simulink library "lib_fuel_converter3"  (Simulink 4.1.1)
values from neighbouring files (symbols this model uses):
  logFlag = 1    [advSACompMaskInit.m]    (also in advSACompMaskInitR13.m)
undefined symbols (not defined in the file or in its folder): air_cp, amb_tmp, cyc_mph, ex_gas_cp, fc_acc_mass, fc_base_mass, fc_c2i_th_cond, fc_c_init_tmp, fc_cl2h_eff, fc_CO2_to_FUELgps, fc_cold, fc_cold_tmp, fc_cp, fc_ct_trq, fc_emisv, fc_ext_sarea, fc_fuel_den, fc_fuel_lhv, fc_h2x_th_cond, fc_h_air_flow, fc_h_cp, fc_h_init_tmp, fc_hood_emisv, fc_hood_sarea, fc_i2x_th_cond, fc_i_init_tmp, fc_inertia, fc_map_spd, fc_map_trq, fc_max_trq, fc_nn_model_name, fc_pwr_scale, fc_spd_scale, fc_trq_scale, fc_tstat, fc_x_init_tmp, fd_ratio, gb_num_init, gb_ratio, generalName, pow, vc_idle_bool, vc_idle_spd, vc_key_on, veh_glider_mass, wh_radius
libraries: lib_fuel_converter3 x4, lib_etc x4, lib_fuel_converter x2, lib_fuel_converter2 x1
(part 6 of 9)

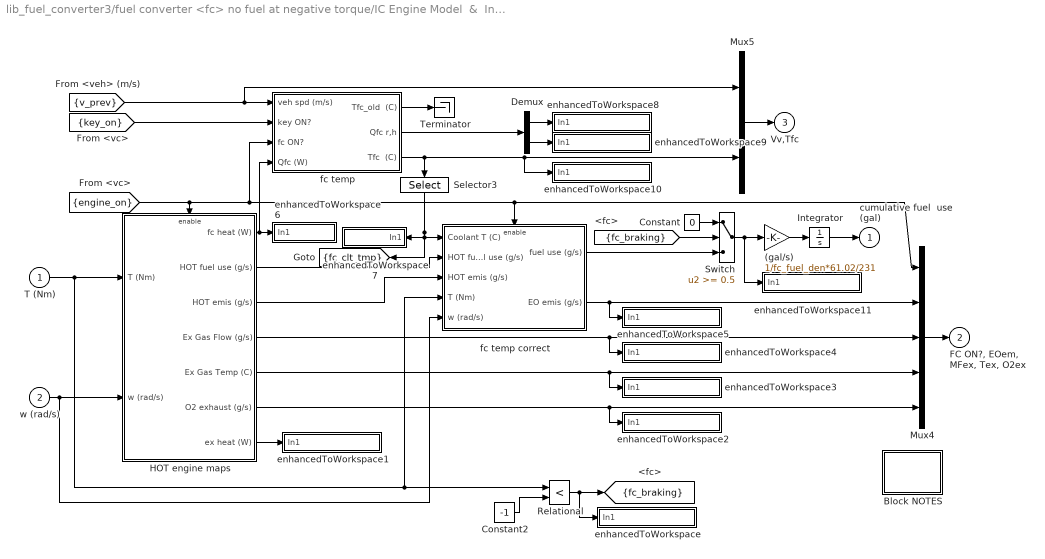
== system lib_fuel_converter3/fuel converter <fc> no fuel at negative torque/IC Engine Model  &  Interface/ic engine model/fuel use and EO emis no fuel used at negative torque ==
  T (Nm) : Inport  Port=1  LatchInput=off
  w (rad/s) : Inport  Port=2  LatchInput=off
  (gal/s) : Gain  Gain=1/fc_fuel_den*61.02/231  Multiplication=Element-wise(K.*u)  SaturateOnIntegerOverflow=on
  Block NOTES : Subsystem
      settings: RTWFcnNameOpts=Auto  RTWFileNameOpts=Auto
      mask Display: disp('Block\nNOTES')
  Constant : Constant  Value=0
  Constant2 : Constant  Value=-1
  Demux : Demux  Outputs=2  BusSelectionMode=off
  "HOT engine maps " : Subsystem  TreatAsAtomicUnit=on
      settings: RTWFcnNameOpts=Auto  RTWFileNameOpts=Auto
  Integrator : Integrator  ExternalReset=none  InitialConditionSource=internal  InitialCondition=0  LimitOutput=off  UpperSaturationLimit=inf  LowerSaturationLimit=-inf  ShowSaturationPort=off  ShowStatePort=off  AbsoluteTolerance=auto
  Mux4 : Mux  Inputs=[1 4 1 1 1]
      settings: DisplayOption=none
  Mux5 : Mux  Inputs=[1 4 ]
      settings: DisplayOption=none
  Relational : RelationalOperator  Operator=<
  Selector3 : Selector  Orientation=down  InputType=Vector  ElementSrc=Internal  Elements=2  RowSrc=Internal  Rows=1  ColumnSrc=Internal  Columns=1  InputPortWidth=4
  Switch : Switch  Threshold=0.5
  Terminator : Terminator
  enhancedToWorkspace : Subsystem  TreatAsAtomicUnit=on  mask(enhancedToWorkspace){generalName=generalName, specificName=braking, logFlag=logFlag}
      mask prompts: generalName "General Name [char-evaluated]"; specificName "Specific Name [char-literal]"; logFlag "Enable flag (1=on,0=off)"
      mask help: A wrapper for the Simulink "To Workspace" block that allows you to evaluate the name of the variable to log to workspace. This is useful to avoid the double logging errors that occur when you pull in two library models that attempt to log to the same variable.
      mask init:
      | enhancedToWsMaker
      settings: CopyFcn=breakLinkCopyFcn  ParentCloseFcn=breakLinkParCloseFcn  RTWFcnNameOpts=Auto  RTWFileNameOpts=Auto
      mask Help:
      | <h2>Enhanced To Workspace Block</h2>
      | <h3>Parameters</h3>
      | <UL>
      | <li><b>General Name:</b> This is the more general name of the variable. Variables are saved to the workspace as <i>generalName_specificName</i>. Note that this is an evaluated variable. If you would like to type in the value directly, it must be surrounded with single quotes. Otherwise you can input the name of a variable containing a char string.</li>
      | <li><b>Specific Name:</b> This is the specific name of the variable. Note that this is input as a char literal (i.e., you don't need quotes).</li>
      | <li><b>Enable Flag:</b> This flag should have the value of 0 or 1. If 0, the variable will not be logged to the workspace. If 1, the variable will be logged. This is done so that variable logging can be turned off to improve speed.</li>
      | </ul>
      | <h3>Overview</h3>
      | <p>The enhanced to workspace block was put together to allow one to dynamically resolve variable names at run time in simulink. This is most powerful when used in conjunction with a masked subsystem to allow multiple instances of that masked subsytem to be used in the same model. The strategy is to set the generalName in the block mask which will allow the block to change the general name for all variable logging on the fly.
      | <h3>Helper Files</h3>
      | <p>Three m-files are required by the enhancedToWorkspace block. These files are located in the &lt; ADVISOR root &gt;/GUI directory :
      | <ul>
      | <li><i>enhancedToWsMaker.m</i> This file runs the mask initialization for the block</li>
      | <li><i>breakLinkCopyFcn.m</i> This file is used by the block callback when the simulink block is copied. It is necessary to break the link to the enhancedToWorkspace similar to the To Workspace block in order for it to be able to configure itself. (Try copying simulink's To Workspace block--it is impossible to make a link)</li>
      | <li><i>breakLinkParCloseFcn.m</i> This file is similar to the breakLinkCopyFcn and is used when a parent system is closed</li>
      | </ul>
      | <hr>
      | 
      | <p>Created 2003-Jan-21, Michael Patrick O'Keefe, NREL</p>
      | 
      | <!--
      | <VARDEF>
      | <H3>var_name</H3>
      | <UL>
      | <LI><B>data type</B> data type here</LI>
      | <LI><B>units</B> units here</LI>
      | <LI><B>vehicle type</B> vehicle type here</LI>
      | <LI><B>description</B> description here</LI>
      | </UL>
      | </VARDEF>
      | -->
      mask Display: disp([generalName,'_',specificName])
  enhancedToWorkspace1 : Subsystem  TreatAsAtomicUnit=on  mask(enhancedToWorkspace){generalName=generalName, specificName=ex_th_pwr, logFlag=logFlag}
      mask prompts: generalName "General Name [char-evaluated]"; specificName "Specific Name [char-literal]"; logFlag "Enable flag (1=on,0=off)"
      mask help: A wrapper for the Simulink "To Workspace" block that allows you to evaluate the name of the variable to log to workspace. This is useful to avoid the double logging errors that occur when you pull in two library models that attempt to log to the same variable.
      mask init:
      | enhancedToWsMaker
      settings: CopyFcn=breakLinkCopyFcn  ParentCloseFcn=breakLinkParCloseFcn  RTWFcnNameOpts=Auto  RTWFileNameOpts=Auto
      mask Help:
      | <h2>Enhanced To Workspace Block</h2>
      | <h3>Parameters</h3>
      | <UL>
      | <li><b>General Name:</b> This is the more general name of the variable. Variables are saved to the workspace as <i>generalName_specificName</i>. Note that this is an evaluated variable. If you would like to type in the value directly, it must be surrounded with single quotes. Otherwise you can input the name of a variable containing a char string.</li>
      | <li><b>Specific Name:</b> This is the specific name of the variable. Note that this is input as a char literal (i.e., you don't need quotes).</li>
      | <li><b>Enable Flag:</b> This flag should have the value of 0 or 1. If 0, the variable will not be logged to the workspace. If 1, the variable will be logged. This is done so that variable logging can be turned off to improve speed.</li>
      | </ul>
      | <h3>Overview</h3>
      | <p>The enhanced to workspace block was put together to allow one to dynamically resolve variable names at run time in simulink. This is most powerful when used in conjunction with a masked subsystem to allow multiple instances of that masked subsytem to be used in the same model. The strategy is to set the generalName in the block mask which will allow the block to change the general name for all variable logging on the fly.
      | <h3>Helper Files</h3>
      | <p>Three m-files are required by the enhancedToWorkspace block. These files are located in the &lt; ADVISOR root &gt;/GUI directory :
      | <ul>
      | <li><i>enhancedToWsMaker.m</i> This file runs the mask initialization for the block</li>
      | <li><i>breakLinkCopyFcn.m</i> This file is used by the block callback when the simulink block is copied. It is necessary to break the link to the enhancedToWorkspace similar to the To Workspace block in order for it to be able to configure itself. (Try copying simulink's To Workspace block--it is impossible to make a link)</li>
      | <li><i>breakLinkParCloseFcn.m</i> This file is similar to the breakLinkCopyFcn and is used when a parent system is closed</li>
      | </ul>
      | <hr>
      | 
      | <p>Created 2003-Jan-21, Michael Patrick O'Keefe, NREL</p>
      | 
      | <!--
      | <VARDEF>
      | <H3>var_name</H3>
      | <UL>
      | <LI><B>data type</B> data type here</LI>
      | <LI><B>units</B> units here</LI>
      | <LI><B>vehicle type</B> vehicle type here</LI>
      | <LI><B>description</B> description here</LI>
      | </UL>
      | </VARDEF>
      | -->
      mask Display: disp([generalName,'_',specificName])
  enhancedToWorkspace10 : Subsystem  TreatAsAtomicUnit=on  mask(enhancedToWorkspace){generalName=generalName, specificName=tmp, logFlag=logFlag}
      mask prompts: generalName "General Name [char-evaluated]"; specificName "Specific Name [char-literal]"; logFlag "Enable flag (1=on,0=off)"
      mask help: A wrapper for the Simulink "To Workspace" block that allows you to evaluate the name of the variable to log to workspace. This is useful to avoid the double logging errors that occur when you pull in two library models that attempt to log to the same variable.
      mask init:
      | enhancedToWsMaker
      settings: CopyFcn=breakLinkCopyFcn  ParentCloseFcn=breakLinkParCloseFcn  RTWFcnNameOpts=Auto  RTWFileNameOpts=Auto
      mask Help:
      | <h2>Enhanced To Workspace Block</h2>
      | <h3>Parameters</h3>
      | <UL>
      | <li><b>General Name:</b> This is the more general name of the variable. Variables are saved to the workspace as <i>generalName_specificName</i>. Note that this is an evaluated variable. If you would like to type in the value directly, it must be surrounded with single quotes. Otherwise you can input the name of a variable containing a char string.</li>
      | <li><b>Specific Name:</b> This is the specific name of the variable. Note that this is input as a char literal (i.e., you don't need quotes).</li>
      | <li><b>Enable Flag:</b> This flag should have the value of 0 or 1. If 0, the variable will not be logged to the workspace. If 1, the variable will be logged. This is done so that variable logging can be turned off to improve speed.</li>
      | </ul>
      | <h3>Overview</h3>
      | <p>The enhanced to workspace block was put together to allow one to dynamically resolve variable names at run time in simulink. This is most powerful when used in conjunction with a masked subsystem to allow multiple instances of that masked subsytem to be used in the same model. The strategy is to set the generalName in the block mask which will allow the block to change the general name for all variable logging on the fly.
      | <h3>Helper Files</h3>
      | <p>Three m-files are required by the enhancedToWorkspace block. These files are located in the &lt; ADVISOR root &gt;/GUI directory :
      | <ul>
      | <li><i>enhancedToWsMaker.m</i> This file runs the mask initialization for the block</li>
      | <li><i>breakLinkCopyFcn.m</i> This file is used by the block callback when the simulink block is copied. It is necessary to break the link to the enhancedToWorkspace similar to the To Workspace block in order for it to be able to configure itself. (Try copying simulink's To Workspace block--it is impossible to make a link)</li>
      | <li><i>breakLinkParCloseFcn.m</i> This file is similar to the breakLinkCopyFcn and is used when a parent system is closed</li>
      | </ul>
      | <hr>
      | 
      | <p>Created 2003-Jan-21, Michael Patrick O'Keefe, NREL</p>
      | 
      | <!--
      | <VARDEF>
      | <H3>var_name</H3>
      | <UL>
      | <LI><B>data type</B> data type here</LI>
      | <LI><B>units</B> units here</LI>
      | <LI><B>vehicle type</B> vehicle type here</LI>
      | <LI><B>description</B> description here</LI>
      | </UL>
      | </VARDEF>
      | -->
      mask Display: disp([generalName,'_',specificName])
  enhancedToWorkspace11 : Subsystem  TreatAsAtomicUnit=on  mask(enhancedToWorkspace){generalName=generalName, specificName=fuel_rate, logFlag=logFlag}
      mask prompts: generalName "General Name [char-evaluated]"; specificName "Specific Name [char-literal]"; logFlag "Enable flag (1=on,0=off)"
      mask help: A wrapper for the Simulink "To Workspace" block that allows you to evaluate the name of the variable to log to workspace. This is useful to avoid the double logging errors that occur when you pull in two library models that attempt to log to the same variable.
      mask init:
      | enhancedToWsMaker
      settings: CopyFcn=breakLinkCopyFcn  ParentCloseFcn=breakLinkParCloseFcn  RTWFcnNameOpts=Auto  RTWFileNameOpts=Auto
      mask Help:
      | <h2>Enhanced To Workspace Block</h2>
      | <h3>Parameters</h3>
      | <UL>
      | <li><b>General Name:</b> This is the more general name of the variable. Variables are saved to the workspace as <i>generalName_specificName</i>. Note that this is an evaluated variable. If you would like to type in the value directly, it must be surrounded with single quotes. Otherwise you can input the name of a variable containing a char string.</li>
      | <li><b>Specific Name:</b> This is the specific name of the variable. Note that this is input as a char literal (i.e., you don't need quotes).</li>
      | <li><b>Enable Flag:</b> This flag should have the value of 0 or 1. If 0, the variable will not be logged to the workspace. If 1, the variable will be logged. This is done so that variable logging can be turned off to improve speed.</li>
      | </ul>
      | <h3>Overview</h3>
      | <p>The enhanced to workspace block was put together to allow one to dynamically resolve variable names at run time in simulink. This is most powerful when used in conjunction with a masked subsystem to allow multiple instances of that masked subsytem to be used in the same model. The strategy is to set the generalName in the block mask which will allow the block to change the general name for all variable logging on the fly.
      | <h3>Helper Files</h3>
      | <p>Three m-files are required by the enhancedToWorkspace block. These files are located in the &lt; ADVISOR root &gt;/GUI directory :
      | <ul>
      | <li><i>enhancedToWsMaker.m</i> This file runs the mask initialization for the block</li>
      | <li><i>breakLinkCopyFcn.m</i> This file is used by the block callback when the simulink block is copied. It is necessary to break the link to the enhancedToWorkspace similar to the To Workspace block in order for it to be able to configure itself. (Try copying simulink's To Workspace block--it is impossible to make a link)</li>
      | <li><i>breakLinkParCloseFcn.m</i> This file is similar to the breakLinkCopyFcn and is used when a parent system is closed</li>
      | </ul>
      | <hr>
      | 
      | <p>Created 2003-Jan-21, Michael Patrick O'Keefe, NREL</p>
      | 
      | <!--
      | <VARDEF>
      | <H3>var_name</H3>
      | <UL>
      | <LI><B>data type</B> data type here</LI>
      | <LI><B>units</B> units here</LI>
      | <LI><B>vehicle type</B> vehicle type here</LI>
      | <LI><B>description</B> description here</LI>
      | </UL>
      | </VARDEF>
      | -->
      mask Display: disp([generalName,'_',specificName])
  enhancedToWorkspace2 : Subsystem  TreatAsAtomicUnit=on  mask(enhancedToWorkspace){generalName=generalName, specificName=o2_flow, logFlag=logFlag}
      mask prompts: generalName "General Name [char-evaluated]"; specificName "Specific Name [char-literal]"; logFlag "Enable flag (1=on,0=off)"
      mask help: A wrapper for the Simulink "To Workspace" block that allows you to evaluate the name of the variable to log to workspace. This is useful to avoid the double logging errors that occur when you pull in two library models that attempt to log to the same variable.
      mask init:
      | enhancedToWsMaker
      settings: CopyFcn=breakLinkCopyFcn  ParentCloseFcn=breakLinkParCloseFcn  RTWFcnNameOpts=Auto  RTWFileNameOpts=Auto
      mask Help:
      | <h2>Enhanced To Workspace Block</h2>
      | <h3>Parameters</h3>
      | <UL>
      | <li><b>General Name:</b> This is the more general name of the variable. Variables are saved to the workspace as <i>generalName_specificName</i>. Note that this is an evaluated variable. If you would like to type in the value directly, it must be surrounded with single quotes. Otherwise you can input the name of a variable containing a char string.</li>
      | <li><b>Specific Name:</b> This is the specific name of the variable. Note that this is input as a char literal (i.e., you don't need quotes).</li>
      | <li><b>Enable Flag:</b> This flag should have the value of 0 or 1. If 0, the variable will not be logged to the workspace. If 1, the variable will be logged. This is done so that variable logging can be turned off to improve speed.</li>
      | </ul>
      | <h3>Overview</h3>
      | <p>The enhanced to workspace block was put together to allow one to dynamically resolve variable names at run time in simulink. This is most powerful when used in conjunction with a masked subsystem to allow multiple instances of that masked subsytem to be used in the same model. The strategy is to set the generalName in the block mask which will allow the block to change the general name for all variable logging on the fly.
      | <h3>Helper Files</h3>
      | <p>Three m-files are required by the enhancedToWorkspace block. These files are located in the &lt; ADVISOR root &gt;/GUI directory :
      | <ul>
      | <li><i>enhancedToWsMaker.m</i> This file runs the mask initialization for the block</li>
      | <li><i>breakLinkCopyFcn.m</i> This file is used by the block callback when the simulink block is copied. It is necessary to break the link to the enhancedToWorkspace similar to the To Workspace block in order for it to be able to configure itself. (Try copying simulink's To Workspace block--it is impossible to make a link)</li>
      | <li><i>breakLinkParCloseFcn.m</i> This file is similar to the breakLinkCopyFcn and is used when a parent system is closed</li>
      | </ul>
      | <hr>
      | 
      | <p>Created 2003-Jan-21, Michael Patrick O'Keefe, NREL</p>
      | 
      | <!--
      | <VARDEF>
      | <H3>var_name</H3>
      | <UL>
      | <LI><B>data type</B> data type here</LI>
      | <LI><B>units</B> units here</LI>
      | <LI><B>vehicle type</B> vehicle type here</LI>
      | <LI><B>description</B> description here</LI>
      | </UL>
      | </VARDEF>
      | -->
      mask Display: disp([generalName,'_',specificName])
  enhancedToWorkspace3 : Subsystem  TreatAsAtomicUnit=on  mask(enhancedToWorkspace){generalName=generalName, specificName=ex_gas_tmp, logFlag=logFlag}
      mask prompts: generalName "General Name [char-evaluated]"; specificName "Specific Name [char-literal]"; logFlag "Enable flag (1=on,0=off)"
      mask help: A wrapper for the Simulink "To Workspace" block that allows you to evaluate the name of the variable to log to workspace. This is useful to avoid the double logging errors that occur when you pull in two library models that attempt to log to the same variable.
      mask init:
      | enhancedToWsMaker
      settings: CopyFcn=breakLinkCopyFcn  ParentCloseFcn=breakLinkParCloseFcn  RTWFcnNameOpts=Auto  RTWFileNameOpts=Auto
      mask Help:
      | <h2>Enhanced To Workspace Block</h2>
      | <h3>Parameters</h3>
      | <UL>
      | <li><b>General Name:</b> This is the more general name of the variable. Variables are saved to the workspace as <i>generalName_specificName</i>. Note that this is an evaluated variable. If you would like to type in the value directly, it must be surrounded with single quotes. Otherwise you can input the name of a variable containing a char string.</li>
      | <li><b>Specific Name:</b> This is the specific name of the variable. Note that this is input as a char literal (i.e., you don't need quotes).</li>
      | <li><b>Enable Flag:</b> This flag should have the value of 0 or 1. If 0, the variable will not be logged to the workspace. If 1, the variable will be logged. This is done so that variable logging can be turned off to improve speed.</li>
      | </ul>
      | <h3>Overview</h3>
      | <p>The enhanced to workspace block was put together to allow one to dynamically resolve variable names at run time in simulink. This is most powerful when used in conjunction with a masked subsystem to allow multiple instances of that masked subsytem to be used in the same model. The strategy is to set the generalName in the block mask which will allow the block to change the general name for all variable logging on the fly.
      | <h3>Helper Files</h3>
      | <p>Three m-files are required by the enhancedToWorkspace block. These files are located in the &lt; ADVISOR root &gt;/GUI directory :
      | <ul>
      | <li><i>enhancedToWsMaker.m</i> This file runs the mask initialization for the block</li>
      | <li><i>breakLinkCopyFcn.m</i> This file is used by the block callback when the simulink block is copied. It is necessary to break the link to the enhancedToWorkspace similar to the To Workspace block in order for it to be able to configure itself. (Try copying simulink's To Workspace block--it is impossible to make a link)</li>
      | <li><i>breakLinkParCloseFcn.m</i> This file is similar to the breakLinkCopyFcn and is used when a parent system is closed</li>
      | </ul>
      | <hr>
      | 
      | <p>Created 2003-Jan-21, Michael Patrick O'Keefe, NREL</p>
      | 
      | <!--
      | <VARDEF>
      | <H3>var_name</H3>
      | <UL>
      | <LI><B>data type</B> data type here</LI>
      | <LI><B>units</B> units here</LI>
      | <LI><B>vehicle type</B> vehicle type here</LI>
      | <LI><B>description</B> description here</LI>
      | </UL>
      | </VARDEF>
      | -->
      mask Display: disp([generalName,'_',specificName])
  enhancedToWorkspace4 : Subsystem  TreatAsAtomicUnit=on  mask(enhancedToWorkspace){generalName=generalName, specificName=ex_gas_flow, logFlag=logFlag}
      mask prompts: generalName "General Name [char-evaluated]"; specificName "Specific Name [char-literal]"; logFlag "Enable flag (1=on,0=off)"
      mask help: A wrapper for the Simulink "To Workspace" block that allows you to evaluate the name of the variable to log to workspace. This is useful to avoid the double logging errors that occur when you pull in two library models that attempt to log to the same variable.
      mask init:
      | enhancedToWsMaker
      settings: CopyFcn=breakLinkCopyFcn  ParentCloseFcn=breakLinkParCloseFcn  RTWFcnNameOpts=Auto  RTWFileNameOpts=Auto
      mask Help:
      | <h2>Enhanced To Workspace Block</h2>
      | <h3>Parameters</h3>
      | <UL>
      | <li><b>General Name:</b> This is the more general name of the variable. Variables are saved to the workspace as <i>generalName_specificName</i>. Note that this is an evaluated variable. If you would like to type in the value directly, it must be surrounded with single quotes. Otherwise you can input the name of a variable containing a char string.</li>
      | <li><b>Specific Name:</b> This is the specific name of the variable. Note that this is input as a char literal (i.e., you don't need quotes).</li>
      | <li><b>Enable Flag:</b> This flag should have the value of 0 or 1. If 0, the variable will not be logged to the workspace. If 1, the variable will be logged. This is done so that variable logging can be turned off to improve speed.</li>
      | </ul>
      | <h3>Overview</h3>
      | <p>The enhanced to workspace block was put together to allow one to dynamically resolve variable names at run time in simulink. This is most powerful when used in conjunction with a masked subsystem to allow multiple instances of that masked subsytem to be used in the same model. The strategy is to set the generalName in the block mask which will allow the block to change the general name for all variable logging on the fly.
      | <h3>Helper Files</h3>
      | <p>Three m-files are required by the enhancedToWorkspace block. These files are located in the &lt; ADVISOR root &gt;/GUI directory :
      | <ul>
      | <li><i>enhancedToWsMaker.m</i> This file runs the mask initialization for the block</li>
      | <li><i>breakLinkCopyFcn.m</i> This file is used by the block callback when the simulink block is copied. It is necessary to break the link to the enhancedToWorkspace similar to the To Workspace block in order for it to be able to configure itself. (Try copying simulink's To Workspace block--it is impossible to make a link)</li>
      | <li><i>breakLinkParCloseFcn.m</i> This file is similar to the breakLinkCopyFcn and is used when a parent system is closed</li>
      | </ul>
      | <hr>
      | 
      | <p>Created 2003-Jan-21, Michael Patrick O'Keefe, NREL</p>
      | 
      | <!--
      | <VARDEF>
      | <H3>var_name</H3>
      | <UL>
      | <LI><B>data type</B> data type here</LI>
      | <LI><B>units</B> units here</LI>
      | <LI><B>vehicle type</B> vehicle type here</LI>
      | <LI><B>description</B> description here</LI>
      | </UL>
      | </VARDEF>
      | -->
      mask Display: disp([generalName,'_',specificName])
  enhancedToWorkspace5 : Subsystem  TreatAsAtomicUnit=on  mask(enhancedToWorkspace){generalName=generalName, specificName=emis_eo, logFlag=logFlag}
      mask prompts: generalName "General Name [char-evaluated]"; specificName "Specific Name [char-literal]"; logFlag "Enable flag (1=on,0=off)"
      mask help: A wrapper for the Simulink "To Workspace" block that allows you to evaluate the name of the variable to log to workspace. This is useful to avoid the double logging errors that occur when you pull in two library models that attempt to log to the same variable.
      mask init:
      | enhancedToWsMaker
      settings: CopyFcn=breakLinkCopyFcn  ParentCloseFcn=breakLinkParCloseFcn  RTWFcnNameOpts=Auto  RTWFileNameOpts=Auto
      mask Help:
      | <h2>Enhanced To Workspace Block</h2>
      | <h3>Parameters</h3>
      | <UL>
      | <li><b>General Name:</b> This is the more general name of the variable. Variables are saved to the workspace as <i>generalName_specificName</i>. Note that this is an evaluated variable. If you would like to type in the value directly, it must be surrounded with single quotes. Otherwise you can input the name of a variable containing a char string.</li>
      | <li><b>Specific Name:</b> This is the specific name of the variable. Note that this is input as a char literal (i.e., you don't need quotes).</li>
      | <li><b>Enable Flag:</b> This flag should have the value of 0 or 1. If 0, the variable will not be logged to the workspace. If 1, the variable will be logged. This is done so that variable logging can be turned off to improve speed.</li>
      | </ul>
      | <h3>Overview</h3>
      | <p>The enhanced to workspace block was put together to allow one to dynamically resolve variable names at run time in simulink. This is most powerful when used in conjunction with a masked subsystem to allow multiple instances of that masked subsytem to be used in the same model. The strategy is to set the generalName in the block mask which will allow the block to change the general name for all variable logging on the fly.
      | <h3>Helper Files</h3>
      | <p>Three m-files are required by the enhancedToWorkspace block. These files are located in the &lt; ADVISOR root &gt;/GUI directory :
      | <ul>
      | <li><i>enhancedToWsMaker.m</i> This file runs the mask initialization for the block</li>
      | <li><i>breakLinkCopyFcn.m</i> This file is used by the block callback when the simulink block is copied. It is necessary to break the link to the enhancedToWorkspace similar to the To Workspace block in order for it to be able to configure itself. (Try copying simulink's To Workspace block--it is impossible to make a link)</li>
      | <li><i>breakLinkParCloseFcn.m</i> This file is similar to the breakLinkCopyFcn and is used when a parent system is closed</li>
      | </ul>
      | <hr>
      | 
      | <p>Created 2003-Jan-21, Michael Patrick O'Keefe, NREL</p>
      | 
      | <!--
      | <VARDEF>
      | <H3>var_name</H3>
      | <UL>
      | <LI><B>data type</B> data type here</LI>
      | <LI><B>units</B> units here</LI>
      | <LI><B>vehicle type</B> vehicle type here</LI>
      | <LI><B>description</B> description here</LI>
      | </UL>
      | </VARDEF>
      | -->
      mask Display: disp([generalName,'_',specificName])
  enhancedToWorkspace6 : Subsystem  TreatAsAtomicUnit=on  mask(enhancedToWorkspace){generalName=generalName, specificName=th_pwr, logFlag=logFlag}
      mask prompts: generalName "General Name [char-evaluated]"; specificName "Specific Name [char-literal]"; logFlag "Enable flag (1=on,0=off)"
      mask help: A wrapper for the Simulink "To Workspace" block that allows you to evaluate the name of the variable to log to workspace. This is useful to avoid the double logging errors that occur when you pull in two library models that attempt to log to the same variable.
      mask init:
      | enhancedToWsMaker
      settings: CopyFcn=breakLinkCopyFcn  ParentCloseFcn=breakLinkParCloseFcn  RTWFcnNameOpts=Auto  RTWFileNameOpts=Auto
      mask Help:
      | <h2>Enhanced To Workspace Block</h2>
      | <h3>Parameters</h3>
      | <UL>
      | <li><b>General Name:</b> This is the more general name of the variable. Variables are saved to the workspace as <i>generalName_specificName</i>. Note that this is an evaluated variable. If you would like to type in the value directly, it must be surrounded with single quotes. Otherwise you can input the name of a variable containing a char string.</li>
      | <li><b>Specific Name:</b> This is the specific name of the variable. Note that this is input as a char literal (i.e., you don't need quotes).</li>
      | <li><b>Enable Flag:</b> This flag should have the value of 0 or 1. If 0, the variable will not be logged to the workspace. If 1, the variable will be logged. This is done so that variable logging can be turned off to improve speed.</li>
      | </ul>
      | <h3>Overview</h3>
      | <p>The enhanced to workspace block was put together to allow one to dynamically resolve variable names at run time in simulink. This is most powerful when used in conjunction with a masked subsystem to allow multiple instances of that masked subsytem to be used in the same model. The strategy is to set the generalName in the block mask which will allow the block to change the general name for all variable logging on the fly.
      | <h3>Helper Files</h3>
      | <p>Three m-files are required by the enhancedToWorkspace block. These files are located in the &lt; ADVISOR root &gt;/GUI directory :
      | <ul>
      | <li><i>enhancedToWsMaker.m</i> This file runs the mask initialization for the block</li>
      | <li><i>breakLinkCopyFcn.m</i> This file is used by the block callback when the simulink block is copied. It is necessary to break the link to the enhancedToWorkspace similar to the To Workspace block in order for it to be able to configure itself. (Try copying simulink's To Workspace block--it is impossible to make a link)</li>
      | <li><i>breakLinkParCloseFcn.m</i> This file is similar to the breakLinkCopyFcn and is used when a parent system is closed</li>
      | </ul>
      | <hr>
      | 
      | <p>Created 2003-Jan-21, Michael Patrick O'Keefe, NREL</p>
      | 
      | <!--
      | <VARDEF>
      | <H3>var_name</H3>
      | <UL>
      | <LI><B>data type</B> data type here</LI>
      | <LI><B>units</B> units here</LI>
      | <LI><B>vehicle type</B> vehicle type here</LI>
      | <LI><B>description</B> description here</LI>
      | </UL>
      | </VARDEF>
      | -->
      mask Display: disp([generalName,'_',specificName])
  enhancedToWorkspace7 : Subsystem  Orientation=left  TreatAsAtomicUnit=on  mask(enhancedToWorkspace){generalName=generalName, specificName=clt_tmp, logFlag=logFlag}
      mask prompts: generalName "General Name [char-evaluated]"; specificName "Specific Name [char-literal]"; logFlag "Enable flag (1=on,0=off)"
      mask help: A wrapper for the Simulink "To Workspace" block that allows you to evaluate the name of the variable to log to workspace. This is useful to avoid the double logging errors that occur when you pull in two library models that attempt to log to the same variable.
      mask init:
      | enhancedToWsMaker
      settings: CopyFcn=breakLinkCopyFcn  ParentCloseFcn=breakLinkParCloseFcn  RTWFcnNameOpts=Auto  RTWFileNameOpts=Auto
      mask Help:
      | <h2>Enhanced To Workspace Block</h2>
      | <h3>Parameters</h3>
      | <UL>
      | <li><b>General Name:</b> This is the more general name of the variable. Variables are saved to the workspace as <i>generalName_specificName</i>. Note that this is an evaluated variable. If you would like to type in the value directly, it must be surrounded with single quotes. Otherwise you can input the name of a variable containing a char string.</li>
      | <li><b>Specific Name:</b> This is the specific name of the variable. Note that this is input as a char literal (i.e., you don't need quotes).</li>
      | <li><b>Enable Flag:</b> This flag should have the value of 0 or 1. If 0, the variable will not be logged to the workspace. If 1, the variable will be logged. This is done so that variable logging can be turned off to improve speed.</li>
      | </ul>
      | <h3>Overview</h3>
      | <p>The enhanced to workspace block was put together to allow one to dynamically resolve variable names at run time in simulink. This is most powerful when used in conjunction with a masked subsystem to allow multiple instances of that masked subsytem to be used in the same model. The strategy is to set the generalName in the block mask which will allow the block to change the general name for all variable logging on the fly.
      | <h3>Helper Files</h3>
      | <p>Three m-files are required by the enhancedToWorkspace block. These files are located in the &lt; ADVISOR root &gt;/GUI directory :
      | <ul>
      | <li><i>enhancedToWsMaker.m</i> This file runs the mask initialization for the block</li>
      | <li><i>breakLinkCopyFcn.m</i> This file is used by the block callback when the simulink block is copied. It is necessary to break the link to the enhancedToWorkspace similar to the To Workspace block in order for it to be able to configure itself. (Try copying simulink's To Workspace block--it is impossible to make a link)</li>
      | <li><i>breakLinkParCloseFcn.m</i> This file is similar to the breakLinkCopyFcn and is used when a parent system is closed</li>
      | </ul>
      | <hr>
      | 
      | <p>Created 2003-Jan-21, Michael Patrick O'Keefe, NREL</p>
      | 
      | <!--
      | <VARDEF>
      | <H3>var_name</H3>
      | <UL>
      | <LI><B>data type</B> data type here</LI>
      | <LI><B>units</B> units here</LI>
      | <LI><B>vehicle type</B> vehicle type here</LI>
      | <LI><B>description</B> description here</LI>
      | </UL>
      | </VARDEF>
      | -->
      mask Display: disp([generalName,'_',specificName])
  enhancedToWorkspace8 : Subsystem  TreatAsAtomicUnit=on  mask(enhancedToWorkspace){generalName=generalName, specificName=r_th_pwr, logFlag=logFlag}
      mask prompts: generalName "General Name [char-evaluated]"; specificName "Specific Name [char-literal]"; logFlag "Enable flag (1=on,0=off)"
      mask help: A wrapper for the Simulink "To Workspace" block that allows you to evaluate the name of the variable to log to workspace. This is useful to avoid the double logging errors that occur when you pull in two library models that attempt to log to the same variable.
      mask init:
      | enhancedToWsMaker
      settings: CopyFcn=breakLinkCopyFcn  ParentCloseFcn=breakLinkParCloseFcn  RTWFcnNameOpts=Auto  RTWFileNameOpts=Auto
      mask Help:
      | <h2>Enhanced To Workspace Block</h2>
      | <h3>Parameters</h3>
      | <UL>
      | <li><b>General Name:</b> This is the more general name of the variable. Variables are saved to the workspace as <i>generalName_specificName</i>. Note that this is an evaluated variable. If you would like to type in the value directly, it must be surrounded with single quotes. Otherwise you can input the name of a variable containing a char string.</li>
      | <li><b>Specific Name:</b> This is the specific name of the variable. Note that this is input as a char literal (i.e., you don't need quotes).</li>
      | <li><b>Enable Flag:</b> This flag should have the value of 0 or 1. If 0, the variable will not be logged to the workspace. If 1, the variable will be logged. This is done so that variable logging can be turned off to improve speed.</li>
      | </ul>
      | <h3>Overview</h3>
      | <p>The enhanced to workspace block was put together to allow one to dynamically resolve variable names at run time in simulink. This is most powerful when used in conjunction with a masked subsystem to allow multiple instances of that masked subsytem to be used in the same model. The strategy is to set the generalName in the block mask which will allow the block to change the general name for all variable logging on the fly.
      | <h3>Helper Files</h3>
      | <p>Three m-files are required by the enhancedToWorkspace block. These files are located in the &lt; ADVISOR root &gt;/GUI directory :
      | <ul>
      | <li><i>enhancedToWsMaker.m</i> This file runs the mask initialization for the block</li>
      | <li><i>breakLinkCopyFcn.m</i> This file is used by the block callback when the simulink block is copied. It is necessary to break the link to the enhancedToWorkspace similar to the To Workspace block in order for it to be able to configure itself. (Try copying simulink's To Workspace block--it is impossible to make a link)</li>
      | <li><i>breakLinkParCloseFcn.m</i> This file is similar to the breakLinkCopyFcn and is used when a parent system is closed</li>
      | </ul>
      | <hr>
      | 
      | <p>Created 2003-Jan-21, Michael Patrick O'Keefe, NREL</p>
      | 
      | <!--
      | <VARDEF>
      | <H3>var_name</H3>
      | <UL>
      | <LI><B>data type</B> data type here</LI>
      | <LI><B>units</B> units here</LI>
      | <LI><B>vehicle type</B> vehicle type here</LI>
      | <LI><B>description</B> description here</LI>
      | </UL>
      | </VARDEF>
      | -->
      mask Display: disp([generalName,'_',specificName])
  enhancedToWorkspace9 : Subsystem  TreatAsAtomicUnit=on  mask(enhancedToWorkspace){generalName=generalName, specificName=h_th_pwr, logFlag=logFlag}
      mask prompts: generalName "General Name [char-evaluated]"; specificName "Specific Name [char-literal]"; logFlag "Enable flag (1=on,0=off)"
      mask help: A wrapper for the Simulink "To Workspace" block that allows you to evaluate the name of the variable to log to workspace. This is useful to avoid the double logging errors that occur when you pull in two library models that attempt to log to the same variable.
      mask init:
      | enhancedToWsMaker
      settings: CopyFcn=breakLinkCopyFcn  ParentCloseFcn=breakLinkParCloseFcn  RTWFcnNameOpts=Auto  RTWFileNameOpts=Auto
      mask Help:
      | <h2>Enhanced To Workspace Block</h2>
      | <h3>Parameters</h3>
      | <UL>
      | <li><b>General Name:</b> This is the more general name of the variable. Variables are saved to the workspace as <i>generalName_specificName</i>. Note that this is an evaluated variable. If you would like to type in the value directly, it must be surrounded with single quotes. Otherwise you can input the name of a variable containing a char string.</li>
      | <li><b>Specific Name:</b> This is the specific name of the variable. Note that this is input as a char literal (i.e., you don't need quotes).</li>
      | <li><b>Enable Flag:</b> This flag should have the value of 0 or 1. If 0, the variable will not be logged to the workspace. If 1, the variable will be logged. This is done so that variable logging can be turned off to improve speed.</li>
      | </ul>
      | <h3>Overview</h3>
      | <p>The enhanced to workspace block was put together to allow one to dynamically resolve variable names at run time in simulink. This is most powerful when used in conjunction with a masked subsystem to allow multiple instances of that masked subsytem to be used in the same model. The strategy is to set the generalName in the block mask which will allow the block to change the general name for all variable logging on the fly.
      | <h3>Helper Files</h3>
      | <p>Three m-files are required by the enhancedToWorkspace block. These files are located in the &lt; ADVISOR root &gt;/GUI directory :
      | <ul>
      | <li><i>enhancedToWsMaker.m</i> This file runs the mask initialization for the block</li>
      | <li><i>breakLinkCopyFcn.m</i> This file is used by the block callback when the simulink block is copied. It is necessary to break the link to the enhancedToWorkspace similar to the To Workspace block in order for it to be able to configure itself. (Try copying simulink's To Workspace block--it is impossible to make a link)</li>
      | <li><i>breakLinkParCloseFcn.m</i> This file is similar to the breakLinkCopyFcn and is used when a parent system is closed</li>
      | </ul>
      | <hr>
      | 
      | <p>Created 2003-Jan-21, Michael Patrick O'Keefe, NREL</p>
      | 
      | <!--
      | <VARDEF>
      | <H3>var_name</H3>
      | <UL>
      | <LI><B>data type</B> data type here</LI>
      | <LI><B>units</B> units here</LI>
      | <LI><B>vehicle type</B> vehicle type here</LI>
      | <LI><B>description</B> description here</LI>
      | </UL>
      | </VARDEF>
      | -->
      mask Display: disp([generalName,'_',specificName])
  fc temp : Subsystem
      settings: RTWFcnNameOpts=Auto  RTWFileNameOpts=Auto
  fc temp correct : Subsystem  TreatAsAtomicUnit=on
      settings: RTWFcnNameOpts=Auto  RTWFileNameOpts=Auto
  cumulative fuel  use (gal) : Outport  Port=1  InitialOutput=0
  "FC ON?, EOem, MFex, Tex, O2ex" : Outport  Port=2  InitialOutput=0
  Vv,Tfc : Outport  Port=3  InitialOutput=0
  tag scope: fc_braking=scoped, fc_clt_tmp=scoped
  wires:
  "HOT engine maps "/6(O2 exhaust (g/s)) -> Mux4/5, enhancedToWorkspace2/1(In1)
  T (Nm)/1 -> "HOT engine maps "/1(T (Nm)), fc temp correct/4(T (Nm)), Relational/1
  w (rad/s)/1 -> fc temp correct/5(w (rad/s)), "HOT engine maps "/2(w (rad/s))
  Mux4/1 -> "FC ON?, EOem, MFex, Tex, O2ex"/1
  Mux5/1 -> Vv,Tfc/1
  [v_prev] -> Mux5/1, fc temp/1(veh spd (m/s))
  "HOT engine maps "/4(Ex Gas Flow (g/s)) -> Mux4/3, enhancedToWorkspace4/1(In1)
  "HOT engine maps "/5(Ex Gas Temp (C)) -> Mux4/4, enhancedToWorkspace3/1(In1)
  Integrator/1 -> cumulative fuel  use (gal)/1
  (gal/s)/1 -> Integrator/1
  "HOT engine maps "/2(HOT fuel use (g/s)) -> fc temp correct/2(HOT fuel use (g/s))
  "HOT engine maps "/3(HOT emis (g/s)) -> fc temp correct/3(HOT emis (g/s))
  fc temp/3(Tfc  (C)) -> Selector3/1, Mux5/2, enhancedToWorkspace10/1(In1)
  fc temp/1(Tfc_old  (C)) -> Terminator/1
  "HOT engine maps "/7(ex heat (W)) -> enhancedToWorkspace1/1(In1)
  Selector3/1 -> [fc_clt_tmp], enhancedToWorkspace7/1(In1), fc temp correct/1(Coolant T (C))
  "HOT engine maps "/1(fc heat (W)) -> fc temp/4(Qfc (W)), enhancedToWorkspace6/1(In1)
  fc temp/2(Qfc r,h) -> Demux/1
  Demux/1 -> enhancedToWorkspace8/1(In1)
  Demux/2 -> enhancedToWorkspace9/1(In1)
  fc temp correct/2(EO emis (g/s)) -> Mux4/2, enhancedToWorkspace5/1(In1)
  [engine_on] -> Mux4/1, fc temp correct/Enable, fc temp/3(fc ON?), "HOT engine maps "/Enable
  [key_on] -> fc temp/2(key ON?)
  Switch/1 -> (gal/s)/1, enhancedToWorkspace11/1(In1)
  Constant/1 -> Switch/1
  fc temp correct/1(fuel use (g/s)) -> Switch/3
  [fc_braking] -> Switch/2
  Constant2/1 -> Relational/2
  Relational/1 -> [fc_braking], enhancedToWorkspace/1(In1)

== system lib_fuel_converter3/fuel converter <fc> no fuel at negative torque/IC Engine Model  &  Interface/ic engine model/help ==
